simulink model "DTC_model"  (R2021a)
settings: Solver=ode23s  StartTime=0.0  StopTime=3  MaxStep=1e-3  RelTol=1e-3
values from neighbouring files (symbols this model uses):
  B = fr    (= 0.6)    [FormulaE_script.m]
  b_psi = [0,1]    [FormulaE_script.m]
  b_s = [-pi/6 pi/6 pi/2 5*pi/6 7*pi/6 3*pi/2]    [FormulaE_script.m]
  b_tau = [-1, 0, 1]    [FormulaE_script.m]
  d = 457*10^-3    (= 0.457)    [FormulaE_script.m]
  J = mass_tot*v_max^2/omega_max^2    (= 41.7698)    [FormulaE_script.m]
  kp_O = par_reg_speed.Kp    [FormulaE_script.m]
  Lks = X_lock_eq/(2*pi*50)    (= 0.00138346649)    [FormulaE_script.m]
  M = X_noload_eq/(2*pi*50)    (= 0.0230577748333)    [FormulaE_script.m]
  mass_tot = 800    [FormulaE_script.m]
  pp = 4    [FormulaE_script.m]
  psi_rd_ref = T_ref./k    [FormulaE_script.m]
  Rr_eq = Rr*Z    (= 0.0289752544097)    [FormulaE_script.m]
  Rs_eq = Rs*Z    (= 0.0289752544097)    [FormulaE_script.m]
  speed_ref = traction(:,1)    [FormulaE_script.m]
  SWT_cmplx = cat(3,[exp(j*4*pi/3) exp(j*5*pi/3) 1 exp(j*pi/3) exp(j*2*pi/3)     exp(j*pi);0 0 0 0 0 0; exp(j*2*pi/3) exp(j*pi) exp(j*4*pi/3)     exp(j*5*pi/3) 1 exp(j*pi/3)],     [exp(j*5*pi/3) 1 exp(j*pi/3) exp(j*2*pi/3) exp(j*pi) exp(j*4*pi/3);     0 0 0 0 0 0; exp(j*pi/3) exp(j*2*pi/3) exp(j*pi) exp(j*4*pi/3)     exp(j*5*pi/3) 1])    [FormulaE_script.m]
  SWT_conf = cat(3,[5 6 1 2 3 4; 7 8 7 8 7 8; 3 4 5 6 1 2],     [6 1 2 3 4 5; 8 7 8 7 8 7; 2 3 4 5 6 1])    [FormulaE_script.m]
  T_ref = d/2*tr*traction(:,2).*40    [FormulaE_script.m]
  Ti_O = kp_O/ki_O    [FormulaE_script.m]
  tr = 1    [FormulaE_script.m]
  V_batt = 800    [FormulaE_script.m]
undefined symbols (not defined in the file or in its folder): magnitude, V_motor
libraries: spsIGBTLib x6, spsVoltageMeasurementLib x3, simulink x2, spsDCVoltageSourceLib x1, spsGroundLib x1, spspowerguiLib x1
settings Model: Creator=secch  LastModifiedBy=secch
settings SolverCC: ZeroCrossAlgorithm=Adaptive  AlgebraicLoopSolver=TrustRegion
settings DebuggingCC: IgnoredZcDiagnostic=none  SFMachineParentedDataDiag=warning

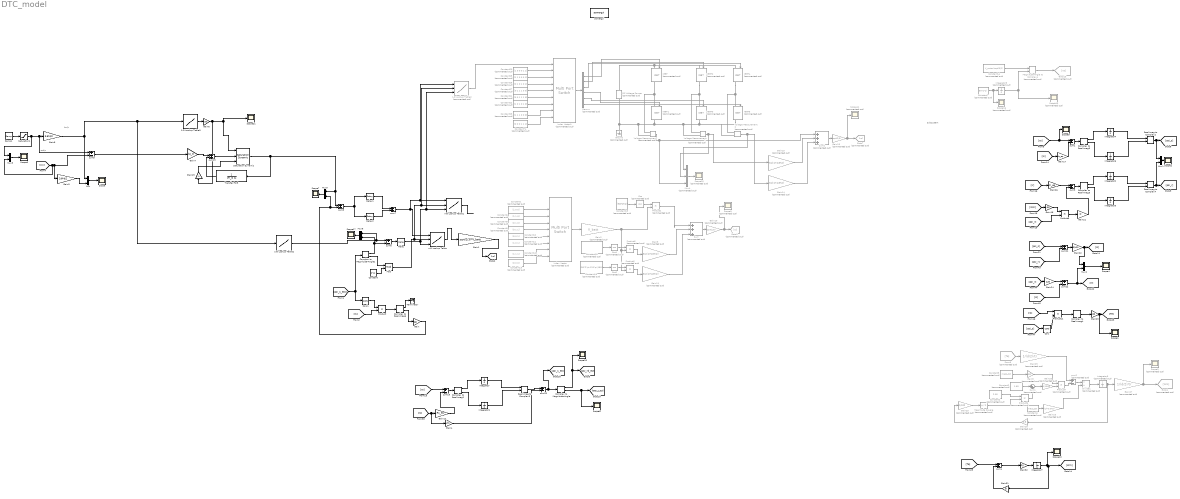
== system DTC_model ==
  note: rad/s
  note: km/h
  note: Subsystem
  1-D Lookup Table2 : Lookup_n-D  NumberOfTableDimensions=1  BreakpointsForDimension1=speed_ref  Table=psi_rd_ref  InternalRulePriority=Speed  RndMeth=Simplest  InputSameDT=on
  1-D Lookup Table3 : Lookup_n-D  NumberOfTableDimensions=1  BreakpointsForDimension1=speed_ref  Table=T_ref  InternalRulePriority=Speed  RndMeth=Simplest  InputSameDT=on
  Complex to Magnitude-Angle : ComplexToMagnitudeAngle
  Complex to Magnitude-Angle1 : ComplexToMagnitudeAngle
  Complex to Real-Imag{2..3,5..6} (4 alike) : ComplexToRealImag
  Complex to Real-Imag4 : ComplexToRealImag  Output=Imag
  Conj : Math  Operator=conj  SaturateOnIntegerOverflow=on
  Conj1 : Math  Operator=conj  SaturateOnIntegerOverflow=on
  Constant : Constant  Value=2*pi
  Constant1 : Constant  Commented=on  Value=[1 0 0]
  Constant10 : Constant  Commented=on  Value=[0 0 1]
  Constant11 : Constant  Commented=on  Value=[1 0 1]
  Constant12 : Constant  Commented=on  Value=[1 1 1]
  Constant13 : Constant  Commented=on  Value=[0 0 0]
  Constant14 : Constant  Commented=on  Value=V_motor*sqrt(3/2)
  Constant15 : Constant  Commented=on  Value=(50*2*pi)
  Constant18 : Constant  Commented=on  Value=(50*2*pi+120*pi/180)
  Constant19 : Constant  Commented=on  Value=(50*2*pi-120*pi/180)
  Constant2 : Constant  Commented=on  Value=2.05
  Constant20 : Constant  Commented=on  Value=[1 0 0 0 1 1]
  Constant21 : Constant  Commented=on  Value=[0 0 1 1 1 0]
  Constant22 : Constant  Commented=on  Value=[1 0 1 0 1 0]
  Constant23 : Constant  Commented=on  Value=[1 1 1 0 0 0]
  Constant24 : Constant  Commented=on  Value=[0 0 0 1 1 1]
  Constant25 : Constant  Commented=on  Value=[1 1 0 0 0 1]
  Constant26 : Constant  Commented=on  Value=[0 1 0 1 0 1]
  Constant27 : Constant  Commented=on  Value=[0 1 1 1 0 0]
  Constant3 : Constant  Commented=on  Value=mass_tot
  Constant4 : Constant  Commented=on  Value=mass_tot
  Constant5 : Constant  Commented=on  Value=1.65
  Constant6 : Constant  Commented=on  Value=[1 1 0]
  Constant7 : Constant  Commented=on  Value=50*2*pi
  Constant8 : Constant  Commented=on  Value=[0 1 0]
  Constant9 : Constant  Commented=on  Value=[0 1 1]
  Cos : Trigonometry  Commented=on  Operator=cos
  Cos1 : Trigonometry  Commented=on  Operator=cos
  Cos2 : Trigonometry  Commented=on  Operator=cos
  DC Voltage Source : spsDCVoltageSourceLib/DC Voltage Source  Commented=on  Amplitude=V_batt  Measurements=None
  Demux : Demux  Commented=on  Outputs=6
  Divide1 : Product  Commented=on  Inputs=*/
  From8 : From  Commented=on  GotoTag=Te
  Gain : Gain  Gain=pp
  Gain1 : Gain  Gain=sqrt(2/3)*V_batt
  Gain10 : Gain  Commented=on  Gain=sqrt(2/3)
  Gain11 : Gain  Commented=on  Gain=exp(1i*4/3*pi)
  Gain12 : Gain  Gain=Rs_eq
  Gain13 : Gain  Commented=on  Gain=sqrt(2/3)
  Gain14 : Gain  Commented=on  Gain=exp(1i*4/3*pi)
  Gain15 : Gain  Commented=on  Gain=exp(1i*2/3*pi)
  Gain16 : Gain  Commented=on  Gain=(1+0.075)
  Gain17 : Gain  Gain=Rs_eq
  Gain18 : Gain  Gain=pp
  Gain19 : Gain  Gain=-1
  Gain2 : Gain  Commented=on  Gain=V_batt
  Gain20 : Gain  Commented=on  Gain=1/1000
  Gain21 : Gain  Gain=1i
  Gain22 : Gain  Gain=1/Lks
  Gain23 : Gain  Gain=pp
  Gain24 : Gain  Gain=1/M
  Gain25 : Gain  Commented=on  Gain=1/100
  Gain26 : Gain  Gain=Rr_eq
  Gain27 : Gain  Commented=on  Gain=1/(d/2)/tr
  Gain28 : Gain  Commented=on  Gain=3.6
  Gain29 : Gain  Commented=on  Gain=1/(d/2)/tr
  Gain3 : Gain  Gain=3.6*d/2
  Gain31 : Gain  Gain=B
  Gain32 : Gain  Gain=1/J
  Gain4 : Gain  Gain=Lks
  Gain5 : Gain  Commented=on  Gain=9.8
  Gain6 : Gain  Gain=100
  Gain7 : Gain  Gain=kp_O
  Gain8 : Gain  Gain=3.6*d/2
  Gain9 : Gain  Commented=on  Gain=exp(1i*2/3*pi)
  Goto1 : Goto  Commented=on  GotoTag=Wm
  Goto13 : Goto  Commented=on  GotoTag=vs
  Goto3 : Goto  Commented=on  GotoTag=vs
  Goto7 : Goto  Commented=on  GotoTag=vs
  Ground : spsGroundLib/Ground  Commented=on  LConnTagsString=a
  IGBT{,1..5} (6 alike) : spsIGBTLib/IGBT  Commented=on  Ron=0.001  Lon=0  Vf=1  Tf=1e-6  Tt=2e-6  IC=0  Rs=1e5  Cs=inf  Measurements=on
  Index Vector : MultiPortSwitch  Commented=on  DataPortOrder=Specify indices  Inputs=1  DataPortIndices={1,2,3,4,5,6,7,8}
  Index Vector1 : MultiPortSwitch  Commented=on  DataPortOrder=Specify indices  Inputs=1  DataPortIndices={1,2,3,4,5,6,7,8}  DiagnosticForDefault=None
  Integrator{,1..3,7} (5 alike) : Integrator
  Integrator4 : Integrator  InitialCondition=1
  Integrator5 : Integrator  Commented=on
  Integrator6 : Integrator  InitialCondition=1
  Integrator8 : Integrator  Commented=on
  Magnitude Square : Math  Commented=on  Operator=magnitude^2  SignedPower=on  RndMeth=Zero  SaturateOnIntegerOverflow=on
  Magnitude-Angle to Complex4 : MagnitudeAngleToComplex  Commented=on
  Mod : Math  Operator=mod  SaturateOnIntegerOverflow=on
  Mux{,1..3,5..6} (6 alike) : Mux  Inputs=2
  Mux4 : Mux  Commented=on  Inputs=3
  Product : Product
  Product{1..2,6..8} (5 alike) : Product  Commented=on
  Product11 : Product
  Product5 : Product
  Ramp1 : simulink/Sources/Ramp  slope=40  start=0  InitialOutput=0
  Real-Imag to Complex2 : RealImagToComplex
  Real-Imag to Complex3 : RealImagToComplex
  Real-Imag to Complex4 : RealImagToComplex
  Relay : Relay  OnSwitchValue=0.001  OffSwitchValue=-0.001
  Relay1 : Relay  OnSwitchValue=1  OffSwitchValue=0
  Relay2 : Relay  OnSwitchValue=0  OffSwitchValue=-1  OnOutputValue=0  OffOutputValue=-1
  Saturation Dynamic : simulink/Discontinuities/Saturation Dynamic  OutMin=[]  OutMax=[]  OutDataTypeStr=Inherit: Same as second input  OutDataType=fixdt(1, 16)  OutScaling=2^-10  DoSatur=off
  Saturation1 : Saturate  UpperLimit=73  LowerLimit=0
  Scope{,1..2,4..8,10,17,20..21} (12 alike) : Scope
  Scope{3,9,11,13,15..16} (6 alike) : Scope  Commented=on
  Sum : Sum  Commented=on  Inputs=|+++
  Sum1 : Sum  Commented=on  Inputs=|++
  Sum2 : Sum  Commented=on  Inputs=|+++
  Terminator : Terminator
  Transfer Fcn5 : TransferFcn  Denominator=[Ti_O 1]
  Voltage Measurement : spsVoltageMeasurementLib/Voltage Measurement  Commented=on  PhasorSimulation=off  OutputType=Complex  PSBequivalent=0
  Voltage Measurement1 : spsVoltageMeasurementLib/Voltage Measurement  Commented=on  PhasorSimulation=off  OutputType=Complex  PSBequivalent=0
  Voltage Measurement2 : spsVoltageMeasurementLib/Voltage Measurement  Commented=on  PhasorSimulation=off  OutputType=Complex  PSBequivalent=0
  n-D Lookup Table : Lookup_n-D  NumberOfTableDimensions=3  BreakpointsForDimension1=b_tau  BreakpointsForDimension2=b_s  BreakpointsForDimension3=b_psi  Table=SWT_cmplx  InterpMethod=Flat  InternalRulePriority=Speed  RndMeth=Simplest  InputSameDT=on
      settings: InputPortMap=u0,u1,u2
  n-D Lookup Table1 : Lookup_n-D  NumberOfTableDimensions=3  BreakpointsForDimension1=b_tau  BreakpointsForDimension2=b_s  BreakpointsForDimension3=b_psi  Table=SWT_conf  InterpMethod=Flat  InternalRulePriority=Speed  RndMeth=Simplest  InputSameDT=on
      settings: InputPortMap=u0,u1,u2
  n-D Lookup Table2 : Lookup_n-D  Commented=on  NumberOfTableDimensions=3  BreakpointsForDimension1=b_tau  BreakpointsForDimension2=b_s  BreakpointsForDimension3=b_psi  Table=SWT_conf  InterpMethod=Flat  InternalRulePriority=Speed  RndMeth=Simplest  InputSameDT=on
      settings: InputPortMap=u0,u1,u2
  powergui : spspowerguiLib/powergui  Priority=1  SimulationMode=Continuous  SampleTime=50e-6  frequency=50  Iterations=50  frequencyindice=0  Pbase=100e6  ErrMax=1e-4  UnitsV=kV  UnitsW=MW  buscounter=0  FunctionMessages=off  echomessages=off  EnableUseOfTLC=off  CurrentSourceSwitches=off  DisableSnubberDevices=off  DisableRonSwitches=off  DisableVfSwitches=off  DisplayEquations=off  AutomaticDiscreteSolvers=off  SolverType=Tustin/Backward Euler (TBE)  Interpol=off  ExternalGateDelay=off  methode=off  Ts=100  x0status=blocks  SPID=on  SwTol=0  HookPort=off  NonlinearTolerance=1e-4  nMaxIteration=100  ContinueOnMaxIteration=off  RestoreLinks=warning  ResistiveCurrentMeasurement=off  Frange=[0:2:500]  Ylog=off  Xlog=on  ShowGrid=off  save=off  variable=ZData  structure=0  ZoomFFT=off  StartTime=0.0  cycles=1  DisplayStyle=1  fundamental=60  FreqAxis=off  MaxFrequency=1000  frequencyindicesteady=1  RmsSteady=1  display=off
  sum{1,4..6,8,19..22} (9 alike) : Sum  Inputs=+-
  sum15 : Sum
  sum2 : Sum  Commented=on  Inputs=+-
  sum3 : Sum  Inputs=-+
  sum7 : Sum
  wires:
  Integrator1/1 -> Real-Imag to Complex3/2
  Integrator/1 -> Real-Imag to Complex3/1
  sum19/1 -> Complex to Real-Imag2/1
  Complex to Real-Imag2/1 -> Integrator/1
  Gain12/1 -> sum19/2
  [vs] -> sum19/1
  [is] -> Gain12/1, Gain4/1
  Complex to Real-Imag2/2 -> Integrator1/1
  Real-Imag to Complex3/1 -> sum20/1
  Gain4/1 -> sum20/2
  sum20/1 -> [psi_s_est], Complex to Magnitude-Angle/1
  Complex to Magnitude-Angle/2 -> Scope8/1, [teta_s_est]
  Complex to Magnitude-Angle/1 -> Scope20/1, [psi_rd_est]
  Divide1/1 -> Integrator5/1
  Gain16/1 -> Divide1/2
  sum2/1 -> Divide1/1
  Gain29/1 -> sum2/1
  From8/1 -> Gain29/1
  Gain5/1 -> Product7/1
  Product7/1 -> sum2/2
  Constant3/1 -> Gain5/1
  Magnitude Square/1 -> Product6/2
  Gain28/1 -> Gain25/1
  Integrator5/1 -> Gain28/1, Gain27/1
  Gain27/1 -> Scope3/1, Goto1/1
  Gain25/1 -> Magnitude Square/1
  Constant2/1 -> Product6/1
  Product6/1 -> Sum1/2
  Constant5/1 -> Sum1/1
  Constant4/1 -> Gain16/1
  Gain23/1 -> Scope1/1, [Te]
  [is] -> Gain17/1
  Real-Imag to Complex2/1 -> Mux1/1, [psi_s]
  [is] -> Product11/1
  sum1/1 -> Complex to Real-Imag5/1
  Gain21/1 -> sum3/2
  [psi_r] -> Product5/2
  [psi_s] -> sum21/1
  Product11/1 -> Complex to Real-Imag4/1
  Gain26/1 -> sum3/1
  [Wm] -> Gain18/1
  Complex to Real-Imag3/2 -> Integrator3/1
  Integrator2/1 -> Real-Imag to Complex4/1
  Product5/1 -> Gain21/1
  sum3/1 -> Complex to Real-Imag3/1
  Integrator6/1 -> Real-Imag to Complex2/2
  Gain17/1 -> sum1/2
  [is] -> sum22/2
  [psi_r] -> sum21/2
  Integrator4/1 -> Real-Imag to Complex2/1
  Gain24/1 -> sum22/1
  Complex to Real-Imag4/1 -> Gain23/1
  [psi_s] -> Conj/1
  Complex to Real-Imag5/1 -> Integrator4/1
  [vs] -> Scope5/1, sum1/1
  Conj/1 -> Product11/2
  sum21/1 -> Gain22/1
  Real-Imag to Complex4/1 -> Mux1/2, [psi_r]
  Complex to Real-Imag5/2 -> Integrator6/1
  Integrator3/1 -> Real-Imag to Complex4/2
  [ir] -> Gain26/1
  [psi_r] -> Gain24/1
  Complex to Real-Imag3/1 -> Integrator2/1
  Gain22/1 -> Mux2/1, [is]
  sum22/1 -> Mux2/2, [ir]
  Gain18/1 -> Product5/1
  Mux1/1 -> Scope2/1
  Mux2/1 -> Scope4/1
  Sum1/1 -> Gain20/1
  Gain20/1 -> Product7/2
  Magnitude-Angle to Complex4/1 -> Goto13/1
  Gain31/1 -> sum4/2
  [Te] -> sum4/1
  sum4/1 -> Gain32/1
  Gain32/1 -> Integrator7/1
  Integrator7/1 -> Gain31/1, [Wm], Scope10/1
  Constant7/1 -> Scope16/1, Integrator8/1
  Constant14/1 -> Magnitude-Angle to Complex4/1
  Integrator8/1 -> Scope13/1, Magnitude-Angle to Complex4/2
  [is] -> Product/2
  Conj1/1 -> Product/1
  [psi_s_est] -> Complex to Magnitude-Angle1/1, Conj1/1
  Product/1 -> Complex to Real-Imag6/1
  Complex to Real-Imag6/1 -> Terminator/1
  Complex to Real-Imag6/2 -> Gain/1
  Complex to Magnitude-Angle1/2 -> Mod/1
  Constant/1 -> Mod/2
  Mod/1 -> n-D Lookup Table2/2, n-D Lookup Table1/2, n-D Lookup Table/2
  Gain1/1 -> [vs]
  sum6/1 -> Relay/1
  Relay/1 -> n-D Lookup Table2/3, n-D Lookup Table1/3, n-D Lookup Table/3
  sum7/1 -> n-D Lookup Table2/1, n-D Lookup Table1/1, n-D Lookup Table/1
  sum8/1 -> Relay2/1, Relay1/1
  Relay2/1 -> sum7/2
  Relay1/1 -> sum7/1
  Gain/1 -> Mux5/2, sum8/2
  Gain8/1 -> 1-D Lookup Table2/1, 1-D Lookup Table3/1, Mux/1
  Transfer Fcn5/1 -> sum15/2
  1-D Lookup Table3/1 -> Gain6/1
  Gain7/1 -> sum15/1
  sum15/1 -> Saturation Dynamic/2
  Saturation Dynamic/1 -> Transfer Fcn5/1, Mux5/1, sum8/1
  Saturation1/1 -> Mux3/1, sum5/1, Gain8/1
  sum5/1 -> Gain7/1
  [Wm] -> Mux3/2, Gain3/1, sum5/2
  Constant1/1 -> Index Vector/2
  Index Vector/1 -> Gain2/1
  Constant6/1 -> Index Vector/3
  Constant8/1 -> Index Vector/4
  Constant9/1 -> Index Vector/5
  Constant10/1 -> Index Vector/6
  Constant11/1 -> Index Vector/7
  Constant12/1 -> Index Vector/8
  Constant13/1 -> Index Vector/9
  Gain10/1 -> Scope9/1, Goto3/1
  Sum/1 -> Gain10/1
  Gain9/1 -> Sum/2
  Gain11/1 -> Sum/3
  Constant15/1 -> Cos/1
  Cos/1 -> Product1/1
  Gain2/1 -> Product8/2, Product2/2, Product1/2
  Product1/1 -> Sum/1
  Cos1/1 -> Product2/1
  Constant18/1 -> Cos1/1
  Constant19/1 -> Cos2/1
  Cos2/1 -> Product8/1
  Product2/1 -> Gain9/1
  Product8/1 -> Gain11/1
  Constant24/1 -> Index Vector1/9
  Constant23/1 -> Index Vector1/8
  Constant22/1 -> Index Vector1/7
  Constant21/1 -> Index Vector1/6
  Constant27/1 -> Index Vector1/5
  Constant26/1 -> Index Vector1/4
  Constant25/1 -> Index Vector1/3
  Constant20/1 -> Index Vector1/2
  Index Vector1/1 -> Demux/1
  Demux/1 -> IGBT/1
  Demux/2 -> IGBT2/1
  Demux/3 -> IGBT4/1
  Demux/4 -> IGBT1/1
  Demux/5 -> IGBT3/1
  Demux/6 -> IGBT5/1
  Voltage Measurement/1 -> Mux4/3, Sum2/1
  Gain14/1 -> Sum2/3
  Gain15/1 -> Sum2/2
  Sum2/1 -> Gain13/1
  Gain13/1 -> Scope11/1, Goto7/1
  Voltage Measurement1/1 -> Mux4/2, Gain15/1
  Voltage Measurement2/1 -> Mux4/1, Gain14/1
  n-D Lookup Table2/1 -> Index Vector1/1
  Mux/1 -> Scope/1
  Gain3/1 -> Mux/2
  Ramp1/1 -> Saturation1/1
  Mux3/1 -> Scope6/1
  Gain19/1 -> Saturation Dynamic/3
  n-D Lookup Table/1 -> Gain1/1
  n-D Lookup Table1/1 -> ?
  Mux4/1 -> Scope15/1
  Gain6/1 -> Gain19/1, Saturation Dynamic/1, Scope21/1
  Mux5/1 -> Scope7/1
  Mux6/1 -> Scope17/1
  1-D Lookup Table2/1 -> Mux6/1, sum6/1
  Complex to Magnitude-Angle1/1 -> Mux6/2, sum6/2
  connections:
  DC Voltage Source/RConn1 -- IGBT4/LConn1 -- IGBT2/LConn1 -- IGBT/LConn1
  IGBT1/RConn1 -- Voltage Measurement1/LConn2 -- Voltage Measurement2/LConn2 -- IGBT5/RConn1 -- IGBT3/RConn1 -- Voltage Measurement/LConn2 -- DC Voltage Source/LConn1 -- Ground/LConn1
  IGBT4/RConn1 -- Voltage Measurement2/LConn1 -- IGBT5/LConn1
  IGBT2/RConn1 -- Voltage Measurement1/LConn1 -- IGBT3/LConn1
  IGBT1/LConn1 -- Voltage Measurement/LConn1 -- IGBT/RConn1
